simulink model "raas_powertrain_model_Copy"  (R2026a)
settings: Solver=ode45  StopTime=474  MaxStep=0.5
undefined symbols (not defined in the file or in its folder): CdA, Crr, eta_drv, eta_regen, grade_rad, mass, rho, wheel_radius_m
settings Model: LastModifiedBy=ASUS USER

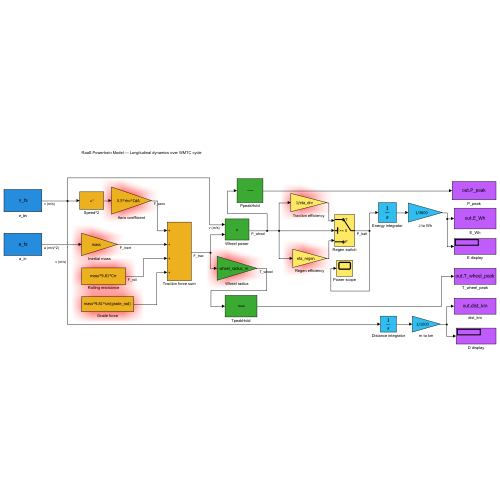
[thumbnail: Simulink's stored preview of the top-level diagram]
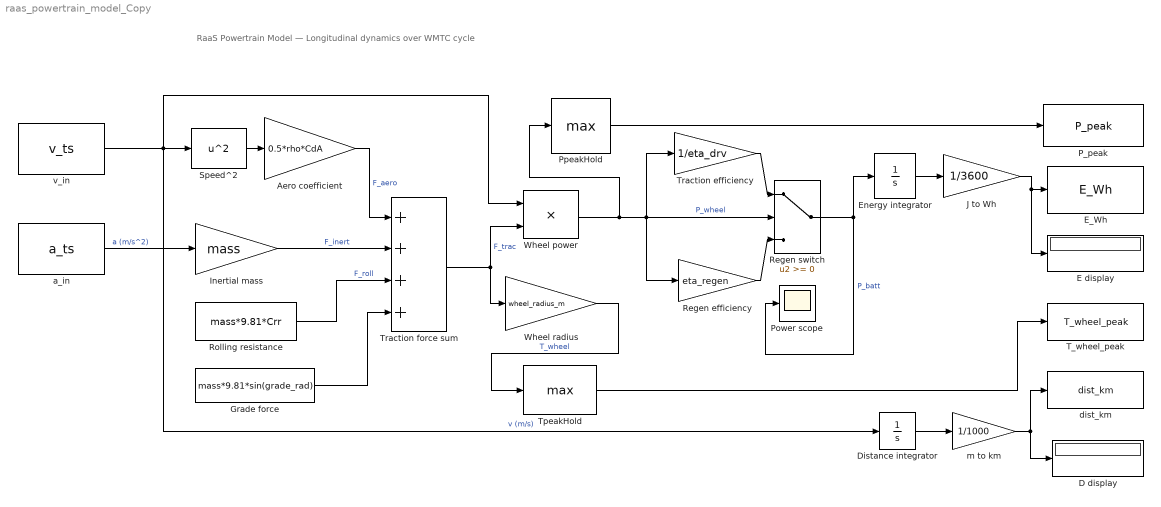
== system raas_powertrain_model_Copy ==
  note: RaaS Powertrain Model — Longitudinal dynamics over WMTC cycle
  Aero coefficient : Gain  Gain=0.5*rho*CdA
  D display : Display
  Distance integrator : Integrator
  E display : Display
  E_Wh : ToWorkspace  VariableName=E_Wh  SampleTime=-1
  Energy integrator : Integrator
  Grade force : Constant  Value=mass*9.81*sin(grade_rad)
  Inertial mass : Gain  Gain=mass
  J to Wh : Gain  Gain=1/3600
  P_peak : ToWorkspace  VariableName=P_peak  SampleTime=-1
  Power scope : Scope
  PpeakHold : MinMax  Function=max
  Regen efficiency : Gain  Gain=eta_regen
  Regen switch : Switch  SaturateOnIntegerOverflow=off  InputSameDT=off
  Rolling resistance : Constant  Value=mass*9.81*Crr
  Speed^2 : Math  Operator=square
  T_wheel_peak : ToWorkspace  VariableName=T_wheel_peak  SampleTime=-1
  TpeakHold : MinMax  Function=max
  Traction efficiency : Gain  Gain=1/eta_drv
  Traction force sum : Sum  Inputs=++++
  Wheel power : Product
  Wheel radius : Gain  Gain=wheel_radius_m
  a_in : FromWorkspace  VariableName=a_ts
  dist_km : ToWorkspace  VariableName=dist_km  SampleTime=-1
  m to km : Gain  Gain=1/1000
  v_in : FromWorkspace  VariableName=v_ts
  wires:
  v_in/1 -> Wheel power/1, Distance integrator/1, Speed^2/1  "v (m/s)"
  Speed^2/1 -> Aero coefficient/1
  a_in/1 -> Inertial mass/1  "a (m/s^2)"
  Rolling resistance/1 -> Traction force sum/3  "F_roll"
  Aero coefficient/1 -> Traction force sum/1  "F_aero"
  Inertial mass/1 -> Traction force sum/2  "F_inert"
  Grade force/1 -> Traction force sum/4
  Traction force sum/1 -> Wheel radius/1, Wheel power/2  "F_trac"
  Wheel radius/1 -> TpeakHold/1  "T_wheel"
  TpeakHold/1 -> T_wheel_peak/1
  Wheel power/1 -> Traction efficiency/1, Regen switch/2, Regen efficiency/1, PpeakHold/1  "P_wheel"
  PpeakHold/1 -> P_peak/1
  Traction efficiency/1 -> Regen switch/1
  Regen efficiency/1 -> Regen switch/3
  Regen switch/1 -> Energy integrator/1, Power scope/1  "P_batt"
  Energy integrator/1 -> J to Wh/1
  J to Wh/1 -> E display/1, E_Wh/1
  Distance integrator/1 -> m to km/1
  m to km/1 -> D display/1, dist_km/1
